simulink model "theta_d"  (R2016a)
settings: Solver=VariableStepAuto  StartTime=0.0  StopTime=600  RelTol=1e-3
values from neighbouring files (symbols this model uses):
  A1 = [X_u+X_T_u X_alpha 0 -g*cos(theta_1) ... (first row only)    [Cesna182_flight_dy.m]
  B1 = [X_de 0 ... (first row only)    [Cesna182_flight_dy.m]
  C1 = [1 0 0 0 ... (first row only)    [Cesna182_flight_dy.m]
  D1 = [0 0 ... (first row only)    [Cesna182_flight_dy.m]
  U_1 = 67.08648    [Cesna182_flight_dy.m]
libraries: simulink x1
settings Model: Creator=felip  LastModifiedBy=felip

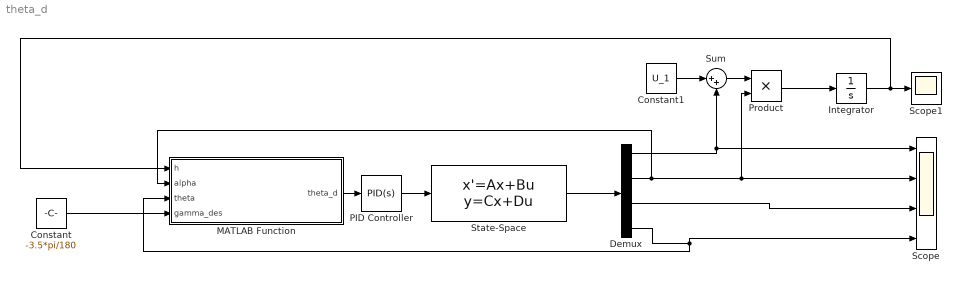
== system theta_d ==
  Constant : Constant  Value=-3.5*pi/180
  Constant1 : Constant  Value=U_1
  Demux : Demux
  Integrator : Integrator  InitialCondition=500
  MATLAB Function : MATLAB Function  TreatAsAtomicUnit=on
  PID Controller : simulink/Continuous/PID Controller  Controller=PID  TimeDomain=Continuous-time  SampleTime=-1  IntegratorMethod=Forward Euler  FilterMethod=Forward Euler  Form=Parallel  UseFilter=on  ControllerParametersSource=internal  P=0  I=-0.00253827581544273  D=0  N=100  InitialConditionSource=internal  InitialConditionForIntegrator=0  InitialConditionForFilter=0  ExternalReset=none  LimitOutput=off  UpperSaturationLimit=inf  LowerSaturationLimit=-inf  LinearizeAsGain=on  AntiWindupMode=none  Kb=1  TrackingMode=off  Kt=1  PParamMin=[]  PParamMax=[]  IParamMin=[]  IParamMax=[]  DParamMin=[]  DParamMax=[]  NParamMin=[]  NParamMax=[]  KbParamMin=[]  KbParamMax=[]  KtParamMin=[]  KtParamMax=[]  POutMin=[]  POutMax=[]  IOutMin=[]  IOutMax=[]  DOutMin=[]  DOutMax=[]  NOutMin=[]  NOutMax=[]  KbOutMin=[]  KbOutMax=[]  KtOutMin=[]  KtOutMax=[]  IntegratorOutMin=[]  IntegratorOutMax=[]  FilterOutMin=[]  FilterOutMax=[]  SumOutMin=[]  SumOutMax=[]  SumI1OutMin=[]  SumI1OutMax=[]  SumI2OutMin=[]  SumI2OutMax=[]  SumI3OutMin=[]  SumI3OutMax=[]  SumDOutMin=[]  SumDOutMax=[]  SaturationOutMin=[]  SaturationOutMax=[]  IntegratorContinuousStateAttributes=''  IntegratorStateMustResolveToSignalObject=off  IntegratorRTWStateStorageClass=Auto  FilterContinuousStateAttributes=''  FilterStateMustResolveToSignalObject=off  FilterRTWStateStorageClass=Auto  DifferentiatorICPrevScaledInput=0  DifferentiatorOutMin=[]  DifferentiatorOutMax=[]
  Product : Product
  Scope : Scope  NumInputPorts=4
  Scope1 : Scope
  State-Space : StateSpace  A=A1  B=B1(:,1)  C=C1  D=D1(:,1)  X0=0
  Sum : Sum  Inputs=|++
  wires:
  State-Space/1 -> Demux/1
  Demux/4 -> MATLAB Function/3(theta), Scope/4
  Demux/3 -> Scope/3
  Constant/1 -> MATLAB Function/4(gamma_des)
  PID Controller/1 -> State-Space/1
  Demux/1 -> Sum/2, Scope/1
  Demux/2 -> MATLAB Function/2(alpha), Product/2, Scope/2
  Product/1 -> Integrator/1
  Integrator/1 -> Scope1/1, MATLAB Function/1(h)
  MATLAB Function/1(theta_d) -> PID Controller/1
  Constant1/1 -> Sum/1
  Sum/1 -> Product/1

== matlab function theta_d/MATLAB Function ==
  data: h input; theta_d output; alpha input; theta input; gamma_des input
function theta_d = fcn(h,alpha,theta,gamma_des)

alpha_des = 2*pi/180;
theta_calc = gamma_des + alpha;

if h< 10
    theta_d  = alpha_des;
else
    theta_d = theta_calc - theta;
end
